simulink model "Assignment2Handout-DESKTOP-ULVHTGD"  (R2021b)
settings: Solver=ode1  StartTime=0.0  StopTime=simulationTime  FixedStep=sampleTime  RelTol=1e-3  EnableMultiTasking=on
InitFcn:
  | cd(fileparts(which(gcs)))
  | 
  | run ./InitModel.m;
StopFcn:
  | run ./DrawPath.m;
values from neighbouring files (symbols this model uses):
  sampleTime = 1e-2    (= 0.01)    [InitModel.m]
  SWA = 3    [InitModel.m]
  vx0 = 80    [InitModel.m]
undefined symbols (not defined in the file or in its folder): vehicleData
settings Model: Creator=arikera  LastModifiedBy=andre
settings SolverCC: AlgebraicLoopSolver=TrustRegion
settings DataIOCC: LimitDataPoints=on  SaveFormat=Array  SignalLoggingSaveFormat=ModelDataLogs  ReturnWorkspaceOutputs=off
settings OptimizationCC: ExpressionDepthLimit=2147483647  LifeSpan=inf
settings DebuggingCC: UnderspecifiedInitializationDetection=Classic  MergeDetectMultiDrivingBlocksExec=none  SolverPrmCheckMsg=warning  FcnCallInpInsideContextMsg=warning  AllowSymbolicDim=off  StateNameClashWarn=warning  SFUnexpectedBacktrackingDiag=warning  SFNoUnconditionalDefaultTransitionDiag=warning  SFExecutionAtInitializationDiag=none  SFMachineParentedDataDiag=warning  ArithmeticOperatorsInVariantConditions=warning
settings HardwareCC: ProdBitPerPointer=32  ProdBitPerSizeT=32  ProdBitPerPtrDiffT=32  ProdLargestAtomicFloat=None  ProdIntDivRoundTo=Undefined  ProdEndianess=Unspecified  ProdWordSize=32  ProdHWDeviceType=32-bit Generic
settings ModelReferenceCC: PropagateSignalLabelsOutOfModel=off
settings SFSimCC: SimUseLocalCustomCode=off  CustomCodeUndefinedFunction=UseInterfaceOnly
settings RTWCC: RTWUseLocalCustomCode=off
settings CodeAppCC: StateflowObjectComments=on
settings GRTTargetCC: TargetLangStandard=C89/C90 (ANSI)  CombineOutputUpdateFcns=off  GRTInterface=on
settings ConfigComp: CovMetricSettings=dw  CovSaveCumulativeToWorkspaceVar=on  CovSaveSingleToWorkspaceVar=on  CovExternalEMLEnable=off  CovSFcnEnable=off

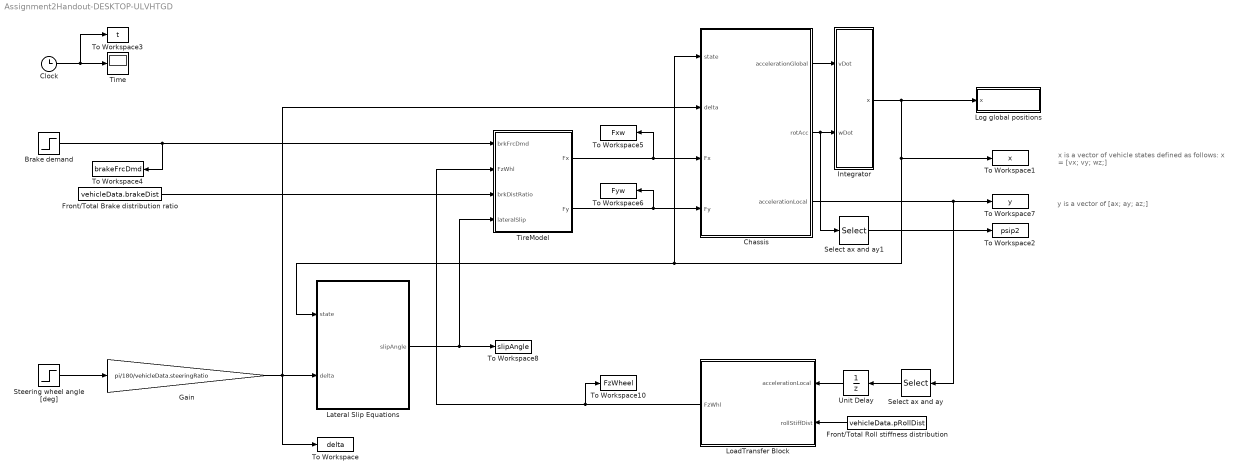
== system Assignment2Handout-DESKTOP-ULVHTGD ==
  note: x is a vector of vehicle states defined as follows:
      | x = [vx; vy; wz;]
  note: y is a vector of [ax; ay; az;]
  Brake demand : Step  Time=3  After=vehicleData.brakeDemand  SampleTime=0
  Chassis : MATLAB Function  TreatAsAtomicUnit=on
  Clock : Clock
  Front/Total Brake distribution ratio : Constant  Value=vehicleData.brakeDist
  Front/Total Roll stiffness distribution : Constant  Value=vehicleData.pRollDist
  Gain : Gain  Gain=pi/180/vehicleData.steeringRatio
  Integrator : Subsystem
  Lateral Slip Equations : MATLAB Function  TreatAsAtomicUnit=on
  LoadTransfer Block : MATLAB Function  TreatAsAtomicUnit=on
  Log global positions : Subsystem
  Select ax and ay : Selector  InputPortWidth=3  IndexOptions=Index vector (dialog)  Indices=[1 2]  OutputSizes=1
  Select ax and ay1 : Selector  InputPortWidth=3  IndexOptions=Index vector (dialog)  Indices=[3]  OutputSizes=1
  Steering wheel angle [deg] : Step  Time=3  After=SWA  SampleTime=0
  Time : Display
  TireModel : Subsystem
  To Workspace : ToWorkspace  VariableName=delta  SampleTime=sampleTime
  To Workspace1 : ToWorkspace  VariableName=x  SampleTime=sampleTime
  To Workspace10 : ToWorkspace  VariableName=FzWheel  SampleTime=sampleTime
  To Workspace2 : ToWorkspace  VariableName=psip2  SampleTime=sampleTime
  To Workspace3 : ToWorkspace  VariableName=t  SampleTime=sampleTime
  To Workspace4 : ToWorkspace  VariableName=brakeFrcDmd  SampleTime=sampleTime
  To Workspace5 : ToWorkspace  VariableName=Fxw  SampleTime=sampleTime
  To Workspace6 : ToWorkspace  VariableName=Fyw  SampleTime=sampleTime
  To Workspace7 : ToWorkspace  VariableName=y  SampleTime=sampleTime
  To Workspace8 : ToWorkspace  VariableName=slipAngle  SampleTime=sampleTime
  Unit Delay : UnitDelay  SampleTime=-1  HasFrameUpgradeWarning=on
  wires:
  LoadTransfer Block/1(FzWhl) -> TireModel/2(FzWhl), To Workspace10/1
  Clock/1 -> To Workspace3/1, Time/1
  Front/Total Roll stiffness distribution/1 -> LoadTransfer Block/2(rollStiffDist)
  Steering wheel angle [deg]/1 -> Gain/1
  Gain/1 -> Lateral Slip Equations/2(delta), Chassis/2(delta), To Workspace/1
  Unit Delay/1 -> LoadTransfer Block/1(accelerationLocal)
  Chassis/1(accelerationGlobal) -> Integrator/1(vDot)
  Chassis/2(rotAcc) -> Select ax and ay1/1, Integrator/2(wDot)
  Select ax and ay/1 -> Unit Delay/1
  Integrator/1(x) -> Log global positions/1(x), Lateral Slip Equations/1(state), Chassis/1(state), To Workspace1/1
  Lateral Slip Equations/1(slipAngle) -> TireModel/4(lateralSlip), To Workspace8/1
  Front/Total Brake distribution ratio/1 -> TireModel/3(brkDistRatio)
  Brake demand/1 -> TireModel/1(brkFrcDmd), To Workspace4/1
  TireModel/1(Fx) -> Chassis/3(Fx), To Workspace5/1
  TireModel/2(Fy) -> Chassis/4(Fy), To Workspace6/1
  Chassis/3(accelerationLocal) -> Select ax and ay/1, To Workspace7/1
  Select ax and ay1/1 -> To Workspace2/1

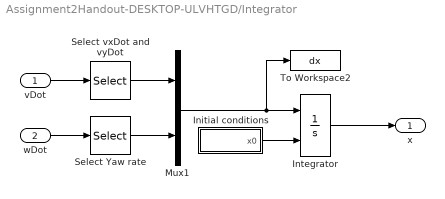
== system Assignment2Handout-DESKTOP-ULVHTGD/Integrator ==
  vDot : Inport
  wDot : Inport  Port=2
  Initial conditions : Subsystem  mask(x0){u0=vx0, v0=0, r0=0}
      mask prompts: u0 "Longitudinal velocity [km/h]"; v0 "Lateral velocity [km/h]"; r0 "Yaw rate [deg/s]"
      mask help: Initial conditions for the simulation
      mask Help:
      | Sets the initial condition for the simulation.
      | 
      | This is a rather simple block that has been made for assignments in the Vehicle Dynamics course (MMF062) at Chalmers since most students enrolled in this course have no prior experience in Simulink.
      | 
      | This block is equivalent to a constant source block with the vector '[u0, v0, r0, ax0, ay0, rDot0]' as the input, where the parameters are as follows:
      | 
      | u0  - Initial longitudinal velocity
      | v0  - Initial lateral velocity
      | r0  - Initial yaw rate
      | 
      | All the parameters are in SI units.
  Integrator : Integrator  InitialConditionSource=external
  Mux1 : Mux  Inputs=2
  Select Yaw rate : Selector  InputPortWidth=3  IndexOptions=Index vector (dialog)  Indices=[3]  OutputSizes=1
  Select vxDot and vyDot : Selector  InputPortWidth=3  IndexOptions=Index vector (dialog)  Indices=[1 2]  OutputSizes=1
  To Workspace2 : ToWorkspace  VariableName=dx  SampleTime=sampleTime
  x : Outport  VectorParamsAs1DForOutWhenUnconnected=off
  wires:
  Select Yaw rate/1 -> Mux1/2
  wDot/1 -> Select Yaw rate/1
  Select vxDot and vyDot/1 -> Mux1/1
  vDot/1 -> Select vxDot and vyDot/1
  Mux1/1 -> To Workspace2/1, Integrator/1
  Initial conditions/1(x0) -> Integrator/2
  Integrator/1 -> x/1

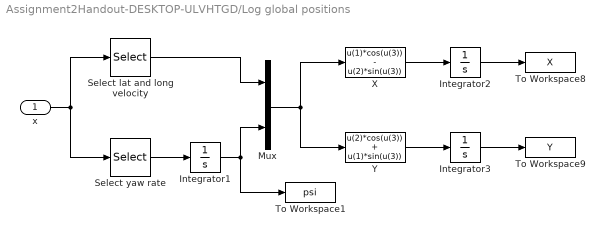
== system Assignment2Handout-DESKTOP-ULVHTGD/Log global positions ==
  x : Inport
  Integrator1 : Integrator
  Integrator2 : Integrator
  Integrator3 : Integrator
  Mux : Mux  Inputs=2
  Select yaw rate : Selector  InputPortWidth=3  IndexOptions=Index vector (dialog)  Indices=3  OutputSizes=1
  Select lat and long velocity : Selector  InputPortWidth=3  IndexOptions=Index vector (dialog)  Indices=[1 2]  OutputSizes=1
  To Workspace1 : ToWorkspace  VariableName=psi  SampleTime=sampleTime
  To Workspace8 : ToWorkspace  VariableName=X  SampleTime=sampleTime
  To Workspace9 : ToWorkspace  VariableName=Y  SampleTime=sampleTime
  X : Fcn  Expr=u(1)*cos(u(3)) - u(2)*sin(u(3))
  Y : Fcn  Expr=u(2)*cos(u(3)) + u(1)*sin(u(3))
  wires:
  Select yaw rate/1 -> Integrator1/1
  Select lat and long velocity/1 -> Mux/1
  Integrator1/1 -> Mux/2, To Workspace1/1
  Mux/1 -> X/1, Y/1
  X/1 -> Integrator2/1
  Y/1 -> Integrator3/1
  x/1 -> Select yaw rate/1, Select lat and long velocity/1
  Integrator2/1 -> To Workspace8/1
  Integrator3/1 -> To Workspace9/1

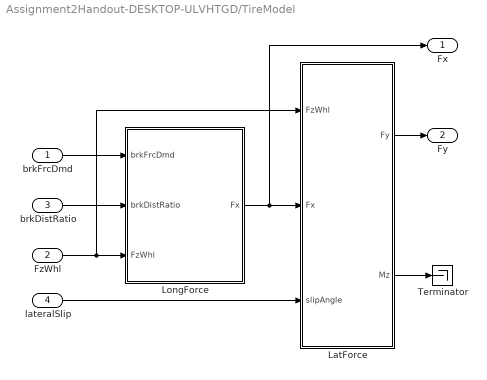
== system Assignment2Handout-DESKTOP-ULVHTGD/TireModel ==
  brkFrcDmd : Inport
  FzWhl : Inport  Port=2
  brkDistRatio : Inport  Port=3
  lateralSlip : Inport  Port=4
  LatForce : MATLAB Function  TreatAsAtomicUnit=on
  LongForce : MATLAB Function  TreatAsAtomicUnit=on
  Terminator : Terminator
  Fx : Outport  VectorParamsAs1DForOutWhenUnconnected=off
  Fy : Outport  Port=2  VectorParamsAs1DForOutWhenUnconnected=off
  wires:
  brkFrcDmd/1 -> LongForce/1(brkFrcDmd)
  brkDistRatio/1 -> LongForce/2(brkDistRatio)
  LongForce/1(Fx) -> LatForce/2(Fx), Fx/1
  LatForce/1(Fy) -> Fy/1
  LatForce/2(Mz) -> Terminator/1
  lateralSlip/1 -> LatForce/3(slipAngle)
  FzWhl/1 -> LatForce/1(FzWhl), LongForce/3(FzWhl)

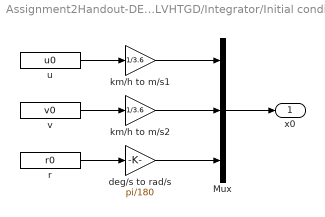
== system Assignment2Handout-DESKTOP-ULVHTGD/Integrator/Initial conditions ==
  Mux : Mux  Inputs=3
  deg/s to rad/s : Gain  Gain=pi/180
  km/h to m/s1 : Gain  Gain=1/3.6
  km/h to m/s2 : Gain  Gain=1/3.6
  r : Constant  Value=r0
  u : Constant  Value=u0
  v : Constant  Value=v0
  x0 : Outport  VectorParamsAs1DForOutWhenUnconnected=off
  wires:
  Mux/1 -> x0/1
  u/1 -> km/h to m/s1/1
  v/1 -> km/h to m/s2/1
  r/1 -> deg/s to rad/s/1
  km/h to m/s1/1 -> Mux/1
  km/h to m/s2/1 -> Mux/2
  deg/s to rad/s/1 -> Mux/3

== matlab function Assignment2Handout-DESKTOP-ULVHTGD/TireModel/LongForce ==
  data: brkFrcDmd input; brkDistRatio input; FzWhl input; Fx output
function Fx  = LongForce(brkFrcDmd,brkDistRatio,FzWhl)
    % Inputs:
    %   FzWhl        - Normal load on tires [N]
    %   brkDistRatio - Front to total brake distribution ratio [-]
    %   brkFrcDmd    - Total brake force demand
    % Outputs:
    %   Fx           - A [2x1] vector with axle longitudinal forces [N]
    
    %%========================DO NOT CHANGE THIS=============================%%
    mu          = 0.8;                                   % Limiting friction coefficient
    FzWhl       = max(FzWhl,[0;0;0;0]);                  % Make sure normal load on wheel does not become negative
    FzFrontAxle = FzWhl(1)+FzWhl(2);                     % Front axle normal load
    FzRearAxle  = FzWhl(3)+FzWhl(4);                     % Rear axle normal load

    %%=======================================================================%%
    % Longitudinal Force
    brkFrcFront = brkDistRatio*brkFrcDmd;                % Braking force on front axle
    brkFrcRear  = brkFrcDmd-brkFrcFront;                 % Braking force on rear axle
    FxFront     = -min(mu*FzFrontAxle,abs(brkFrcFront)); % Limit maximum value
    FxRear      = -min(mu*FzRearAxle,abs(brkFrcRear));   % Limit maximum value
    Fx          = [FxFront;FxRear];
    %%=======================================================================%%
end

== matlab function Assignment2Handout-DESKTOP-ULVHTGD/TireModel/LatForce ==
  data: FzWhl input; Fx input; slipAngle input; Fy output; vehicleData parameter; Mz output
function [Fy,Mz]  = LatForce(FzWhl,Fx,slipAngle,vehicleData)
%#codegen
    %   © CASTER / MMF062
    %   Created: 2019-11-18
    % Inputs:
    %   FzWhl      - Normal load on tires [N]
    %   Fx         - Longitudinal force vector [N]
    %   slipAngle  - Slip angle vector [rad]
    % Outputs:
    %   Fy         - A [2x1] vector with axle lateral forces [N]
    %   Mz         - Dummy value for StrWhlTrq [Nm]
    %
    %%========================DO NOT CHANGE THIS=============================%%
    c0          = vehicleData.c0;                       % Tyre stiffness parameter
    c1          = vehicleData.c1;                       % Tyre stiffness parameter
    mu          = 0.8;

    FzWhl       = max(FzWhl,[0;0;0;0]);                 % Limit minimum value
    FzFrontAxle = FzWhl(1)+FzWhl(2);                    % Front axle normal load
    FzRearAxle  = FzWhl(3)+FzWhl(4);                    % Rear axle normal load
    FzAxle      = [FzFrontAxle;FzRearAxle];
    %%=======================================================================%%
    
    % Axle stiffness calculation (keep in mind that the tyre data is for one
    % wheel and not an axle)
    maxLatForce = [0;0];
    
    % Fx could have been limited when it is calculated
    if (Fx(1)^2>=(mu*FzFrontAxle)^2)
        Cf             = 1e-3;                             % Solving the numerical problems
        maxLatForce(1) = 0;
    else
        %%=======================================================================%%
       Cf = (c0*FzWhl(1)+c1*FzWhl(1)^2)+ (c0*FzWhl(2)+c1*FzWhl(2)^2);%Per axle;                             % Front cornering stiffness
        %Cf = (c0*(FzFrontAxle)+c1*FzFrontAxle^2);%Per axle;                             % Front cornering stiffness

        %%=======================================================================%%
        
        maxLatForce(1) = sqrt((mu*FzAxle(1))^2-Fx(1)^2);   % Friction circle
        
        %%=============================FOR TASK 4================================%%
        % Combined Slip
        % Cf             =  ??;
        %%=======================================================================%%
    end
    
    if (Fx(2)^2>=(mu*FzRearAxle)^2)
        Cr             = 1e-3;                             % Solving the numerical problems
        maxLatForce(2) = 0;
    else
        %%=======================================================================%%
        Cr = (c0*FzWhl(3)+c1*FzWhl(3)^2)+ (c0*FzWhl(4)+c1*FzWhl(4)^2);                             % Rear cornering stiffness
        %Cr =    (c0*(FzRearAxle)+c1*FzRearAxle^2);                          % Rear cornering stiffness

        %%=======================================================================%%
        
        maxLatForce(2) = sqrt((mu*FzAxle(2))^2-Fx(2)^2);   % Friction circle
        
        %%=============================FOR TASK 4================================%%
        % Combined Slip
        % Cr             =  ??;
        %%=======================================================================%%
    end
    
    % Lateral force
    CAxle = [Cf;Cr];
    Fy    =  [-CAxle(1)*tan(slipAngle(1)); -CAxle(2)*tan(slipAngle(2))];
    
    %%========================DO NOT CHANGE THIS=============================%%
    Fy    = min(maxLatForce,abs(Fy)).*sign(Fy);            % Saturation of Fy to sqrt(Fz^2-Fx^2)
    %%=======================================================================%%
    % Self-aligning moment
    A  = -0.001;
    C  = 0.4;
    Mz = A*Fy(1)*C;
    %%=======================================================================%%
end

== matlab function Assignment2Handout-DESKTOP-ULVHTGD/Chassis ==
  data: state input; accelerationGlobal output; rotAcc output; delta input; Fx input; Fy input; accelerationLocal output; vehicleData parameter
function [accelerationGlobal,rotAcc,accelerationLocal] = VehDynModel(state,delta,Fx,Fy,vehicleData)
    %   © CASTER / MMF062
    %   Created: 2019-11-18
    % Inputs:
    %   state  - state vector
    %   delta  - steering wheel angle [rad]
    %   Fx     - Vector of forces from the wheels in x-direction
    %   Fy     - Vector of forces from the wheels in y-direction
    % Outputs: 
    %   accelerationGlobal  - global vehicle acceleration
    %                         [vxDot; vyDot; vzDot]
    %   rotAcc              - vector of vehicle rotational accelerations
    %                         [wx; wy; wz]
    %   accelerationLocal   - local vehicle acceleration 
    %                         [ax; ay; az]
    %
    % ----- Parameters -----
    %%========================DO NOT CHANGE THIS=============================%%
    m         = vehicleData.m;            % Mass of vehicle
    J         = vehicleData.J;
    lf        = vehicleData.lf;           % Distance of CoG from front axle
    lr        = vehicleData.lr;           % Distance of CoG from rear axle
    
    % State vector
    vx        = state(1);
    vy        = state(2);
    wz        = state(3);
    
    %%=======================================================================%%
    % Equations of motion  -
    % ---------------------------------DONT FORGET TO TAKE THE WHEEL
    % COORDINATE SYSTEM INTO ACCOUNT, FOR EXAMPLE FY IS FY IN WHEEL
    
    %From wheel coordinates to vehicle coordinates, eq 1.6 page 83
    Ffw = [Fx(1);Fy(1)]; %Force front wheel coordinate
    Ffv = [cos(delta) -sin(delta); sin(delta) cos(delta)]*Ffw; %Force front vehicle coordinate
    
    Fxv = [Ffv(1);Fx(2)];
    Fyv = [Ffv(2);Fy(2)];
    vxDot     = (vy*wz*m + Fxv(1) + Fxv(2))/m;       % Derivative of longtidunial velocity 
    vyDot     = (-vx*wz*m + Fyv(1) + Fyv(2))/m;       % Derivative of lateral velocity
    wzDot     = (lf*Fyv(1) - lr*Fyv(2))/vehicleData.J;       % Derivative of yaw rotational velocity
    %%========================DO NOT CHANGE THIS=============================%%
    vzDot     = 0;
    wxDot     = 0;
    wyDot     = 0;
      

    % Accelerations
    accelerationGlobal = [vxDot;vyDot;vzDot];
    ax                 = vxDot-wz*vy; 
    ay                 = vyDot+wz*vx;
    az                 = 0;
    accelerationLocal  = [ax;ay;az];

    % Rotational accelerations
    rotAcc             = [wxDot;wyDot;wzDot];
    %%=======================================================================%%
end


% end of file

== matlab function Assignment2Handout-DESKTOP-ULVHTGD/Lateral Slip Equations ==
  data: state input; slipAngle output; delta input; vehicleData parameter
function slipAngle   = LateralSlip(state,delta,vehicleData) 
    %   © CASTER / MMF062
    %   Created: 2019-11-18
    % Inputs:
    %   state     - State vector
    %   delta     - steering wheel angle [rad]
    % Outputs:
    %   slipangle - A [2x1] vector containing the slipratio(0-1) for each axle [-]
    %
    %%========================DO NOT CHANGE THIS=============================%%
    % ----- Parameters -----
    % State vector
    vx = state(1);
    vy = state(2);
    wz = state(3);
    lf = vehicleData.lf;           % Distance of CoG from front axle
    lr = vehicleData.lr;           % Distance of CoG from rear axle
    % Preventing vx from being zero 
    vx = max(abs(vx),3);

    %%=======================================================================%%
    % Slip equations
    alphaf    = atan2(vy+lf*wz,vx)-delta;%*vehicleData.steeringRatio;%atan2((vy+lf*wz)/vx-delta);   %  Front lateral tire slip 
    alphar    = atan2(vy-lr*wz,vx);%atan((vy-lr*wz)/vx);   %  Rear lateral tire slip
    
    slipAngle = [alphaf; alphar];  % Slip angle vector
    %%=======================================================================%%

end

% end of file

== matlab function Assignment2Handout-DESKTOP-ULVHTGD/LoadTransfer Block ==
  data: accelerationLocal input; rollStiffDist input; vehicleData parameter; FzWhl output
function FzWhl  = RollModel(accelerationLocal,rollStiffDist,vehicleData)
    %   © CASTER / MMF062
    %   Created: 2019-11-18
    % Inputs: 
    %   accelerationLocal - vector of vehicle loacl acceleration [ax; ay; az;]
    %   rollStiffDist     - Roll stiffness distribution 0-1 on the front axle [-]
    % Outputs: 
    %   FzWhl             - vector of tyre normal forces [N]
    %
    % ----- Parameters -----
    
    %%========================DO NOT CHANGE THIS=============================%%
    h       = vehicleData.h;            % Center of gravity height
    g       = vehicleData.g;            % Acceleration due to gravity
    m       = vehicleData.m;            % Mass of vehicle
    cRoll   = vehicleData.cw;           % Total roll stiffness
    h1      = vehicleData.hrcf;         % Front roll center height
    h2      = vehicleData.hrcr;         % Rear roll center height
    L       = vehicleData.L;            % Wheelbase
    lf      = vehicleData.lf;           % Distance of CoG from front axle
    lr      = vehicleData.lr;           % Distance of CoG from rear axle
    dh      = h-(h1*lr+h2*lf)/L;        % Height of CoG from roll axis
    w       = vehicleData.w;            % Vehicle track width
    cfRoll  = cRoll*rollStiffDist;      % Front roll stiffness
    crRoll  = cRoll-cfRoll;             % Rear roll stiffness

    %%=======================================================================%%
    % Longitudinal and lateral acceleration
    ax      = accelerationLocal(1); 
    ay      = accelerationLocal(2);
    
    % Longitudinal load transfer (should be modified by students for tasks 3 and 4.)
    deltaFflzLong = m*-ax*h/(2*L);                      % Front left
    deltaFfrzLong = m*-ax*h/(2*L);                      % Front right
    deltaFrlzLong = m*ax*h/(2*L);                      % Rear left
    deltaFrrzLong = m*ax*h/(2*L);                      % Rear right  

    % Lateral load transfer (should be modified by students for tasks 3 and 4.)
    deltaFflzLat  = m*-ay*(h1*lr/(L*w)+dh/w*cfRoll/cRoll);    % Front left
    deltaFfrzLat  = m*ay*(h1*lr/(L*w)+dh/w*cfRoll/cRoll) ;    % Front right
    deltaFrlzLat  = m*-ay*(h2*lr/(L*w)+dh/w*crRoll/cRoll);    % Rear left
    deltaFrrzLat  = m*ay*(h2*lr/(L*w)+dh/w*crRoll/cRoll);     % Rear right
    %%=======================================================================%%

    % Collecting longitudinal and lateral load transfers
    deltaFzLong   = [deltaFflzLong; deltaFfrzLong; deltaFrlzLong; deltaFrrzLong];
    deltaFzLat    = [deltaFflzLat; deltaFfrzLat; deltaFrlzLat; deltaFrrzLat];

    % Total load transfer
    dFz           = deltaFzLong+deltaFzLat;
    FzStatic      = m*g/2/L*[lr; lr; lf; lf];
    FzWhl         = FzStatic+dFz;
    
    %%=======================FOR DRIVING SIMULATOR===========================%%
    % Switch off the load transfer if needed.
    %FzWhl         = FzStatic;
    
    %%========================DO NOT CHANGE THIS=============================%%
    % Wheel lift-off scenario. This is not really *handling* wheel lift-off,
    % but rather making sure the simulation does not crash in the event of
    % wheel lift-off. Solution may still be incorrect. Handling wheel lift-off
    % is not straight forward. So this simulation model is not good for cases
    % with excessive or frequent wheel lift-off.
    if any(FzWhl<=0)
        FzWhl(FzWhl<1e-3) = 1e-3;
    end
end


function Ku = CalcKu(lf1,m)
c0 = 30.7;
c1 = -0.00235;
g = 9.81;
F_fz = m*g*(1-lf1)/2; %Per wheel
F_rz = m*g*lf1/2; %Per wheel
L_f = CAR.L*lf1;
L_r = CAR.L*(1-lf1);

Cf = 2*(c0*F_fz+c1*F_fz^2);%Per axle
Cr = 2*(c0*F_rz+c1*F_rz^2);%Per axle 
Ku = (Cr*L_r-Cf*L_f)/(Cf*Cr*CAR.L);
end
% end of file
